simulink model "stp"  (R2016b)
settings: Solver=VariableStepAuto  StartTime=0.0  StopTime=10.0  RelTol=1e-3
undefined symbols (not defined in the file): Ad, Ad2, Bd2, Cd, Kd
settings Model: Creator=arq  LastModifiedBy=arq

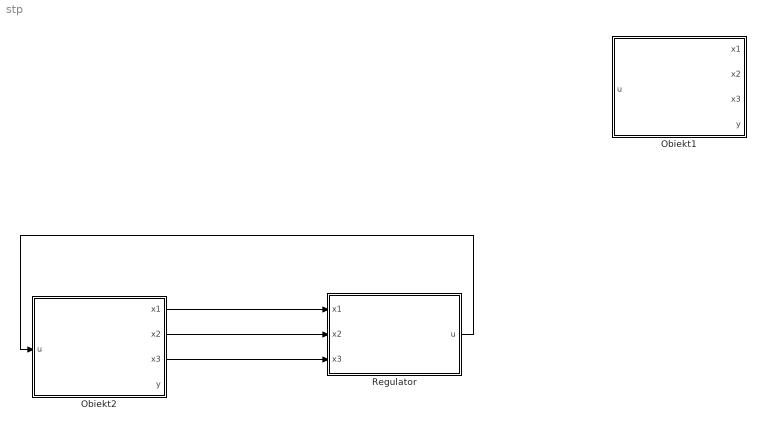
== system stp ==
  Obiekt1 : Subsystem
  "Obiekt2 " : Subsystem
  Regulator : Subsystem
  wires:
  "Obiekt2 "/1(x1) -> Regulator/1(x1)
  "Obiekt2 "/2(x2) -> Regulator/2(x2)
  "Obiekt2 "/3(x3) -> Regulator/3(x3)
  Regulator/1(u) -> "Obiekt2 "/1(u)

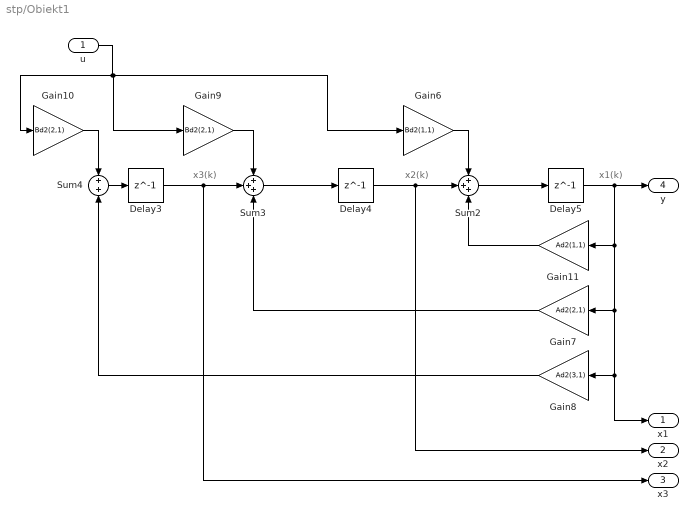
== system stp/Obiekt1 ==
  note: x3(k)
  note: x2(k)
  note: x1(k)
  u : Inport
  Delay3 : Delay  DelayLength=1  InitialCondition=0
  Delay4 : Delay  DelayLength=1  InitialCondition=0
  Delay5 : Delay  DelayLength=1  InitialCondition=0
  Gain10 : Gain  Gain=Bd2(2,1)
  Gain11 : Gain  Gain=Ad2(1,1)
  Gain6 : Gain  Gain=Bd2(1,1)
  Gain7 : Gain  Gain=Ad2(2,1)
  Gain8 : Gain  Gain=Ad2(3,1)
  Gain9 : Gain  Gain=Bd2(2,1)
  Sum2 : Sum  Inputs=3
  Sum3 : Sum  Inputs=3
  Sum4 : Sum  Inputs=2
  x1 : Outport
  x2 : Outport  Port=2
  x3 : Outport  Port=3
  y : Outport  Port=4
  wires:
  Delay5/1 -> y/1, x1/1, Gain8/1, Gain7/1, Gain11/1
  u/1 -> Gain10/1, Gain9/1, Gain6/1
  Delay4/1 -> x2/1, Sum2/2
  Sum2/1 -> Delay5/1
  Sum3/1 -> Delay4/1
  Delay3/1 -> x3/1, Sum3/2
  Gain11/1 -> Sum2/3
  Gain7/1 -> Sum3/3
  Gain8/1 -> Sum4/2
  Sum4/1 -> Delay3/1
  Gain6/1 -> Sum2/1
  Gain9/1 -> Sum3/1
  Gain10/1 -> Sum4/1

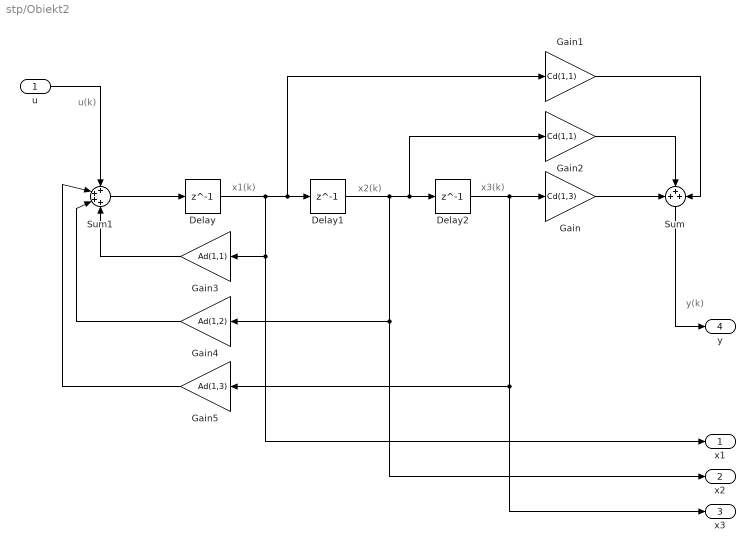
== system stp/Obiekt2  ==
  note: u(k)
  note: x3(k)
  note: x2(k)
  note: x1(k)
  note: y(k)
  u : Inport
  Delay : Delay  DelayLength=1  InitialCondition=0
  Delay1 : Delay  DelayLength=1  InitialCondition=0
  Delay2 : Delay  DelayLength=1  InitialCondition=0
  Gain : Gain  Gain=Cd(1,3)
  Gain1 : Gain  Gain=Cd(1,1)
  Gain2 : Gain  Gain=Cd(1,1)
  Gain3 : Gain  Gain=Ad(1,1)
  Gain4 : Gain  Gain=Ad(1,2)
  Gain5 : Gain  Gain=Ad(1,3)
  Sum : Sum  Inputs=3
  Sum1 : Sum  Inputs=4
  x1 : Outport
  x2 : Outport  Port=2
  x3 : Outport  Port=3
  y : Outport  Port=4
  wires:
  Delay/1 -> x1/1, Gain3/1, Gain1/1, Delay1/1
  Delay1/1 -> x2/1, Gain4/1, Gain2/1, Delay2/1
  Delay2/1 -> Gain5/1, x3/1, Gain/1
  Gain/1 -> Sum/1
  Gain2/1 -> Sum/2
  Gain1/1 -> Sum/3
  Sum1/1 -> Delay/1
  u/1 -> Sum1/1
  Gain3/1 -> Sum1/4
  Gain4/1 -> Sum1/3
  Gain5/1 -> Sum1/2
  Sum/1 -> y/1

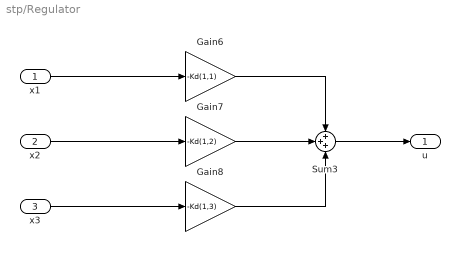
== system stp/Regulator ==
  x1 : Inport
  x2 : Inport  Port=2
  x3 : Inport  Port=3
  Gain6 : Gain  Gain=-Kd(1,1)
  Gain7 : Gain  Gain=-Kd(1,2)
  Gain8 : Gain  Gain=-Kd(1,3)
  Sum3 : Sum  Inputs=+++
  u : Outport
  wires:
  Gain6/1 -> Sum3/1
  Gain7/1 -> Sum3/2
  Gain8/1 -> Sum3/3
  Sum3/1 -> u/1
  x1/1 -> Gain6/1
  x2/1 -> Gain7/1
  x3/1 -> Gain8/1
